simulink model "A3"  (R2016b)
settings: Solver=VariableStepAuto  StartTime=0.0  StopTime=3  RelTol=1e-3
libraries: simulink x1
settings Model: Creator=jonathankirchman  LastModifiedBy=jonathankirchman

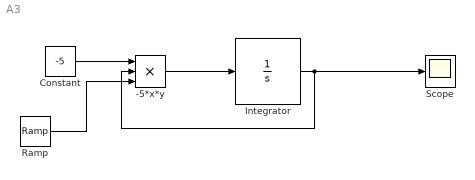
== system A3 ==
  "-5*x*y " : Product  Inputs=3
  Constant : Constant  Value=-5
  Integrator : Integrator  InitialCondition=3
  Ramp : simulink/Sources/Ramp  slope=1  start=0  X0=0
  Scope : Scope
  wires:
  Constant/1 -> "-5*x*y "/1
  "-5*x*y "/1 -> Integrator/1
  Integrator/1 -> Scope/1, "-5*x*y "/2
  Ramp/1 -> "-5*x*y "/3
